simulink model "Dc"  (R2020b)
settings: Solver=VariableStepAuto  StartTime=0.0  StopTime=10.0  RelTol=1e-3
model workspace (MAT data in the model file):
  J = 3.2284e-06
  K = 0.0274
  L = 2.75e-06
  R = 4
  b = 3.5077e-06
settings Model: Creator=user  LastModifiedBy=user

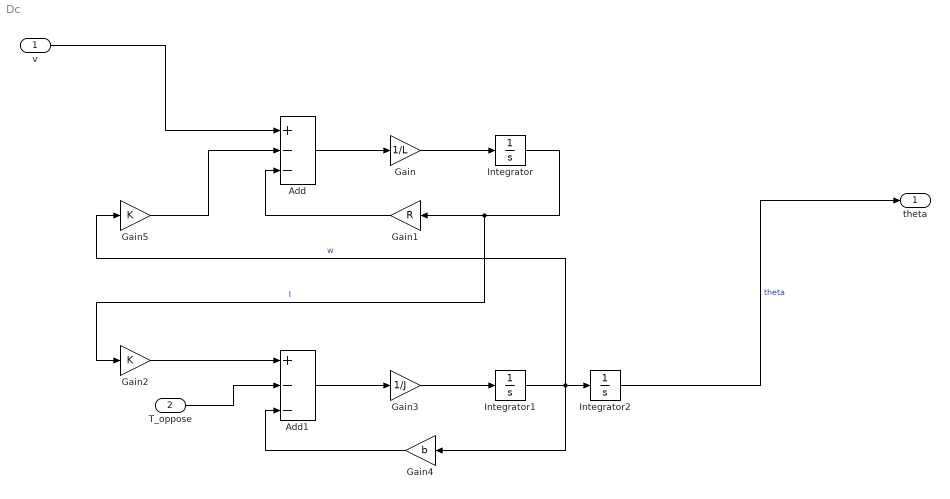
== system Dc ==
  v : Inport  OutDataTypeStr=double  PortDimensions=1  SampleTime=0
  T_oppose : Inport  Port=2  OutDataTypeStr=double  PortDimensions=1
  Add : Sum  Inputs=+--
  Add1 : Sum  Inputs=+--
  Gain : Gain  Gain=1/L
  Gain1 : Gain  Gain=R
  Gain2 : Gain  Gain=K
  Gain3 : Gain  Gain=1/J
  Gain4 : Gain  Gain=b
  Gain5 : Gain  Gain=K
  Integrator : Integrator
  Integrator1 : Integrator
  Integrator2 : Integrator
  theta : Outport  OutDataTypeStr=double  PortDimensions=1  SampleTime=0
  wires:
  Integrator1/1 -> Integrator2/1, Gain5/1, Gain4/1  "w"
  Gain1/1 -> Add/3
  v/1 -> Add/1
  Gain2/1 -> Add1/1
  Integrator/1 -> Gain1/1, Gain2/1  "I"
  Gain4/1 -> Add1/3
  Gain3/1 -> Integrator1/1
  Add/1 -> Gain/1
  Integrator2/1 -> theta/1  "theta"
  Gain5/1 -> Add/2
  T_oppose/1 -> Add1/2
  Gain/1 -> Integrator/1
  Add1/1 -> Gain3/1
